simulink model "EC_control"  (R2023b)
settings: configuration reference "ctrl_tsk_conf" (kept outside this file)
settings Model: DataDictionary=fmuGenerationDictionay.sldd  ModifiedByFormat=Third Equation Ltd  Creator=Third Equation Ltd  LastModifiedBy=Third Equation Ltd
settings ConfigSetRef: SourceName=ctrl_tsk_conf

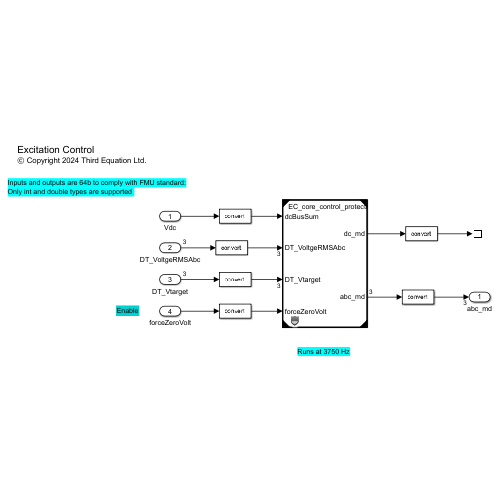
[thumbnail: Simulink's stored preview of the top-level diagram]
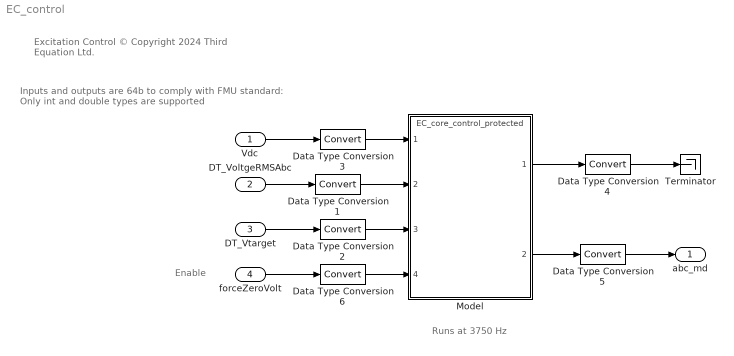
== system EC_control ==
  note: Enable
  note: Excitation Control
      | © Copyright 2024 Third Equation Ltd.
  note: Inputs and outputs are 64b to comply with FMU standard:
      | Only int and double types are supported
  note: Runs at 3750 Hz
  Vdc : Inport  OutDataTypeStr=double  PortDimensions=1
  DT_VoltgeRMSAbc : Inport  Port=2  OutDataTypeStr=double  Unit=V  PortDimensions=3
  DT_Vtarget : Inport  Port=3  OutDataTypeStr=double  Unit=V  PortDimensions=3
  forceZeroVolt : Inport  Port=4  OutDataTypeStr=int32  Unit=V  PortDimensions=1
  Data Type Conversion{1..6} (6 alike) : DataTypeConversion  SaturateOnIntegerOverflow=off  RndMeth=Floor
  Model : ModelReference  ModelNameDialog=EC_core_control_protected.slxp  ModelReferenceVersion=1.40  CopyOfModelProtected=on
  Terminator : Terminator
  abc_md : Outport  OutDataTypeStr=double  PortDimensions=3
  wires:
  Model/1 -> Data Type Conversion4/1
  Model/2 -> Data Type Conversion5/1
  DT_Vtarget/1 -> Data Type Conversion2/1
  DT_VoltgeRMSAbc/1 -> Data Type Conversion1/1
  Vdc/1 -> Data Type Conversion3/1
  Data Type Conversion1/1 -> Model/2
  Data Type Conversion2/1 -> Model/3
  Data Type Conversion3/1 -> Model/1
  Data Type Conversion4/1 -> Terminator/1
  Data Type Conversion5/1 -> abc_md/1
  Data Type Conversion6/1 -> Model/4
  forceZeroVolt/1 -> Data Type Conversion6/1
